simulink model "SF009A_DutyCycThermProtn"  (R2013b)
settings: Solver=FixedStepDiscrete  SolverMode=SingleTasking  StartTime=0.0  StopTime=1  FixedStep=0.1  RelTol=1e-3
undefined symbols (not defined in the file): AbsltTThermLimCnt, ARCHGLBPRM_100MILLISEC_SEC_F32, CTRLRANDCUTFLT_CNT_U08, CTRLRTFLT_CNT_U08, CUTFLT_CNT_U08, DITHERMLIM_MOTNWTMTR_F32, DutyCycExcddCnt, DutyCycThermProtnAbsltCtrlTTblX, DutyCycThermProtnAbsltCtrlTTqTblY, DutyCycThermProtnAbsltCuTTblX, DutyCycThermProtnAbsltCuTTqTblY, DutyCycThermProtnAbsltMotVelBreakPt, DutyCycThermProtnAbsltTTqSlewHiLim, DutyCycThermProtnAbsltTTqSlewLoLim, DutyCycThermProtnCtrlT, DutyCycThermProtnCtrlTSeln, DutyCycThermProtnDutyCycFildThd, DutyCycThermProtnIgnOffCtrlEna, DutyCycThermProtnIgnOffMsgWaitTi, DutyCycThermProtnLstTblValNonStall, DutyCycThermProtnLstTblValStall, DutyCycThermProtnMotPrTSeln, DutyCycThermProtnMplr1NonStallTblY, DutyCycThermProtnMplr1StallTblY, DutyCycThermProtnMplr2NonStallTblY, DutyCycThermProtnMplr2StallTblY, DutyCycThermProtnMplr3NonStallTblY, DutyCycThermProtnMplr3StallTblY, DutyCycThermProtnMplr4NonStallTblY, DutyCycThermProtnMplr4StallTblY, DutyCycThermProtnMplr5NonStallTblY, DutyCycThermProtnMplr5StallTblY, DutyCycThermProtnMplr6NonStallTblY, DutyCycThermProtnMplr6StallTblY, DutyCycThermProtnMplrTblX, DutyCycThermProtnMplrTSeln, DutyCycThermProtnSlowFilTSeln, DutyCycThermProtnThermLoadLimTblX, DutyCycThermProtnThermLoadLimTblY, DutyCycThermProtnTqCmdSlewDwn, DutyCycThermProtnTqCmdSlewUp, FILVALMIN_ULS_F32, IGNTIOFFTHD_CNT_F32, NODEBSTEP_CNT_U16, NtcSts1, NvmGetErrSts1, ONEPERC_ULS_F32, TAU3_SEC_F32, TAU4_SEC_F32, TAU5_SEC_F32, TAU6_SEC_F32, THERMLOADLIMTBLIDX_ULS_U08
libraries: FixdToFloat x13, Fil x12, simulink x11, NxtrLim x10, NxtrMath x8, FloatToFixd x6, NxtrMax x6, NxtrMin x4, NxtrAbslt x2, NxtrNvM x1
(part 4 of 6)

== system SF009A_DutyCycThermProtn/DutyCycThermProtn/DutyCycThermProtnPer1/TemperatureSelection/Mult36T_DiagcStsLimdTPrfmncDisabled ==
  MotMagT : Inport
  MotWidgT : Inport  Port=2
  Action Port : ActionPort  ActionType=else
  Calibration2 : Constant  RequirementInfo="{'linktype_rmi_doors' '0000a52a (/E-STEER Core/SubSystem Specifications/Application Functions/SF009A Thermal Duty Cycle Protection)' '#SF009A_144' 'true' 'REQ:  SF009A_144' '' } %GIDa_f0f24eda_9e7b_4d73_b7e4_5f6aa894dd73"  Value=DutyCycThermProtnMotPrTSeln
  CopyRight2 : Subsystem  Description=|  mask(Copyright Information){none=on}
      | Copyright info block.                                               
      |                                                                     
      | Place copyright information at the top of every subsystem in design.
      mask prompts: none "No parameters"
      mask help: Place copyright information at the top of every subsystem in design.
      mask Display:
      | NxtrConf = 'Nexteer Confidential';
      | 
      | sys = bdroot; %handle for the current model ("system")
      | first = get_param(sys,'Created');
      | first = first(end-3:end);  %year is last four digits
      | 
      | last = get_param(sys,'LastModifiedDate');
      | if isempty(last)
      |     last = datestr(now,'yyyy');
      | else
      |     last = last(end-3:end);
      | end
      | 
      | if strcmp(first,last)
      |     fprintf('%s -- Copyright %s Nexteer',NxtrConf,first)
      | else
      |     fprintf('%s -- %s%s- %s Nexteer',NxtrConf,char(169),first,last)
      | end
  If4 : If  RequirementInfo="{'linktype_rmi_doors' '0000a52a (/E-STEER Core/SubSystem Specifications/Application Functions/SF009A Thermal Duty Cycle Protection)' '#SF009A_144' 'true' 'REQ:  SF009A_144' '' } %GIDa_9a47a2e9_7f28_43d1_84f7_9c3425e558ba"  IfExpression=u1
  Merge4 : Merge  RequirementInfo="{'linktype_rmi_doors' '0000a52a (/E-STEER Core/SubSystem Specifications/Application Functions/SF009A Thermal Duty Cycle Protection)' '#SF009A_144' 'true' 'REQ:  SF009A_144' '' } %GIDa_e830a63c_d6ec_4209_a7ba_269af8b2217d"
  MotPrTSelnDisabled : Subsystem  RequirementInfo="{'linktype_rmi_doors' '0000a52a (/E-STEER Core/SubSystem Specifications/Application Functions/SF009A Thermal Duty Cycle Protection)' '#SF009A_144' 'true' 'REQ:  SF009A_144' '' } %GIDa_b554413f_6212_4f00_8e7a_d2a51ebc8c5c"  TreatAsAtomicUnit=on
  MotPrTSelnEnabled : Subsystem  RequirementInfo="{'linktype_rmi_doors' '0000a52a (/E-STEER Core/SubSystem Specifications/Application Functions/SF009A Thermal Duty Cycle Protection)' '#SF009A_144' 'true' 'REQ:  SF009A_144' '' } %GIDa_5495cb55_f8bc_4002_89d3_d2e432b2479b"  TreatAsAtomicUnit=on
  Mult36Temp : Outport
  wires:
  MotPrTSelnEnabled/1(Mult36) -> Merge4/1
  MotPrTSelnDisabled/1(Mult36) -> Merge4/2
  Calibration2/1 -> If4/1
  MotMagT/1 -> MotPrTSelnEnabled/1(MotMagT)
  MotWidgT/1 -> MotPrTSelnDisabled/1(MotWidgT)
  If4/1 -> MotPrTSelnEnabled/Action
  If4/2 -> MotPrTSelnDisabled/Action
  Merge4/1 -> Mult36Temp/1  "Mult36"

== system SF009A_DutyCycThermProtn/DutyCycThermProtn/DutyCycThermProtnPer1/TemperatureSelection/Mult36T_DiagcStsLimdTPrfmncEnabled ==
  Action Port : ActionPort  ActionType=then
  Calibration4 : Constant  RequirementInfo="{'linktype_rmi_doors' '0000a52a (/E-STEER Core/SubSystem Specifications/Application Functions/SF009A Thermal Duty Cycle Protection)' '#SF009A_144' 'true' 'REQ:  SF009A_144' '' } %GIDa_3ed4d287_d822_4a57_b7ce_3b57540e0243"  Value=DutyCycThermProtnCtrlT
  CopyRight2 : Subsystem  Description=|  mask(Copyright Information){none=on}
      | Copyright info block.                                               
      |                                                                     
      | Place copyright information at the top of every subsystem in design.
      mask prompts: none "No parameters"
      mask help: Place copyright information at the top of every subsystem in design.
      mask Display:
      | NxtrConf = 'Nexteer Confidential';
      | 
      | sys = bdroot; %handle for the current model ("system")
      | first = get_param(sys,'Created');
      | first = first(end-3:end);  %year is last four digits
      | 
      | last = get_param(sys,'LastModifiedDate');
      | if isempty(last)
      |     last = datestr(now,'yyyy');
      | else
      |     last = last(end-3:end);
      | end
      | 
      | if strcmp(first,last)
      |     fprintf('%s -- Copyright %s Nexteer',NxtrConf,first)
      | else
      |     fprintf('%s -- %s%s- %s Nexteer',NxtrConf,char(169),first,last)
      | end
  Mult36Temp : Outport
  wires:
  Calibration4/1 -> Mult36Temp/1

== system SF009A_DutyCycThermProtn/DutyCycThermProtn/DutyCycThermProtnPer1/TempratureLimiting/CopyRight2 ==

== system SF009A_DutyCycThermProtn/DutyCycThermProtn/DutyCycThermProtnPer1/TempratureLimiting/SetCtrlrAndCuTFltNtc ==
  Action Port : ActionPort  ActionType=then
  Constant23 : Constant  RequirementInfo="{'linktype_rmi_doors' '0000a52a (/E-STEER Core/SubSystem Specifications/Application Functions/SF009A Thermal Duty Cycle Protection)' '#SF009A_248' 'true' 'REQ:  SF009A_248' '' } %GIDa_eecd097f_77ad_4a7b_bdb8_19b5b9b4f39b"  Value=CTRLRANDCUTFLT_CNT_U08
  CopyRight2 : Subsystem  Description=|  mask(Copyright Information){none=on}
      | Copyright info block.                                               
      |                                                                     
      | Place copyright information at the top of every subsystem in design.
      mask prompts: none "No parameters"
      mask help: Place copyright information at the top of every subsystem in design.
      mask Display:
      | NxtrConf = 'Nexteer Confidential';
      | 
      | sys = bdroot; %handle for the current model ("system")
      | first = get_param(sys,'Created');
      | if(isempty(first))
      |     first = datestr(now,'yyyy');
      | else
      |     first = first(end-3:end);  %year is last four digits
      | end
      | 
      | last = get_param(sys,'LastModifiedDate');
      | if isempty(last)
      |     last = datestr(now,'yyyy');
      | else
      |     last = last(end-3:end);
      | end
      | 
      | if strcmp(first,last)
      |     fprintf('%s -- Copyright %s Nexteer',NxtrConf,first)
      | else
      |     fprintf('%s -- %s%s- %s Nexteer',NxtrConf,char(169),first,last)
      | end
  Enumerated Constant7 : simulink/Sources/Enumerated Constant  RequirementInfo="{'linktype_rmi_doors' '0000a52a (/E-STEER Core/SubSystem Specifications/Application Functions/SF009A Thermal Duty Cycle Protection)' '#SF009A_248' 'true' 'REQ:  SF009A_248' '' } %GIDa_403c372b_2528_42cf_824a_3c84739cf9bb"  OutDataTypeStr=Enum: NtcSts1  Value=NtcSts1.NTCSTS_FAILD  SampleTime=inf
  Out1 : Outport
  Out2 : Outport  Port=2
  wires:
  Constant23/1 -> Out1/1
  Enumerated Constant7/1 -> Out2/1

== system SF009A_DutyCycThermProtn/DutyCycThermProtn/DutyCycThermProtnPer1/TempratureLimiting/SetCtrlrTFltNtc ==
  Action Port : ActionPort  ActionType=elseif
  Constant25 : Constant  RequirementInfo="{'linktype_rmi_doors' '0000a52a (/E-STEER Core/SubSystem Specifications/Application Functions/SF009A Thermal Duty Cycle Protection)' '#SF009A_248' 'true' 'REQ:  SF009A_248' '' } %GIDa_45d14f2e_33e7_442d_980c_33b708f78f49"  Value=CTRLRTFLT_CNT_U08
  CopyRight2 : Subsystem  Description=|  mask(Copyright Information){none=on}
      | Copyright info block.                                               
      |                                                                     
      | Place copyright information at the top of every subsystem in design.
      mask prompts: none "No parameters"
      mask help: Place copyright information at the top of every subsystem in design.
      mask Display:
      | NxtrConf = 'Nexteer Confidential';
      | 
      | sys = bdroot; %handle for the current model ("system")
      | first = get_param(sys,'Created');
      | if(isempty(first))
      |     first = datestr(now,'yyyy');
      | else
      |     first = first(end-3:end);  %year is last four digits
      | end
      | 
      | last = get_param(sys,'LastModifiedDate');
      | if isempty(last)
      |     last = datestr(now,'yyyy');
      | else
      |     last = last(end-3:end);
      | end
      | 
      | if strcmp(first,last)
      |     fprintf('%s -- Copyright %s Nexteer',NxtrConf,first)
      | else
      |     fprintf('%s -- %s%s- %s Nexteer',NxtrConf,char(169),first,last)
      | end
  Enumerated Constant13 : simulink/Sources/Enumerated Constant  RequirementInfo="{'linktype_rmi_doors' '0000a52a (/E-STEER Core/SubSystem Specifications/Application Functions/SF009A Thermal Duty Cycle Protection)' '#SF009A_248' 'true' 'REQ:  SF009A_248' '' } %GIDa_05e09b87_7e7f_4e95_9fb1_18c3f562049e"  OutDataTypeStr=Enum: NtcSts1  Value=NtcSts1.NTCSTS_FAILD  SampleTime=inf
  Out1 : Outport
  Out2 : Outport  Port=2
  wires:
  Enumerated Constant13/1 -> Out2/1
  Constant25/1 -> Out1/1

== system SF009A_DutyCycThermProtn/DutyCycThermProtn/DutyCycThermProtnPer1/TempratureLimiting/SetCuTFltNtc ==
  Action Port : ActionPort  ActionType=elseif
  Constant27 : Constant  RequirementInfo="{'linktype_rmi_doors' '0000a52a (/E-STEER Core/SubSystem Specifications/Application Functions/SF009A Thermal Duty Cycle Protection)' '#SF009A_248' 'true' 'REQ:  SF009A_248' '' } %GIDa_5abe4f1d_a9ab_402f_b899_5b241470b6cc"  Value=CUTFLT_CNT_U08
  CopyRight2 : Subsystem  Description=|  mask(Copyright Information){none=on}
      | Copyright info block.                                               
      |                                                                     
      | Place copyright information at the top of every subsystem in design.
      mask prompts: none "No parameters"
      mask help: Place copyright information at the top of every subsystem in design.
      mask Display:
      | NxtrConf = 'Nexteer Confidential';
      | 
      | sys = bdroot; %handle for the current model ("system")
      | first = get_param(sys,'Created');
      | if(isempty(first))
      |     first = datestr(now,'yyyy');
      | else
      |     first = first(end-3:end);  %year is last four digits
      | end
      | 
      | last = get_param(sys,'LastModifiedDate');
      | if isempty(last)
      |     last = datestr(now,'yyyy');
      | else
      |     last = last(end-3:end);
      | end
      | 
      | if strcmp(first,last)
      |     fprintf('%s -- Copyright %s Nexteer',NxtrConf,first)
      | else
      |     fprintf('%s -- %s%s- %s Nexteer',NxtrConf,char(169),first,last)
      | end
  Enumerated Constant15 : simulink/Sources/Enumerated Constant  RequirementInfo="{'linktype_rmi_doors' '0000a52a (/E-STEER Core/SubSystem Specifications/Application Functions/SF009A Thermal Duty Cycle Protection)' '#SF009A_248' 'true' 'REQ:  SF009A_248' '' } %GIDa_13f324ce_9b74_4823_8d4c_43ce25139662"  OutDataTypeStr=Enum: NtcSts1  Value=NtcSts1.NTCSTS_FAILD  SampleTime=inf
  Out1 : Outport
  Out2 : Outport  Port=2
  wires:
  Constant27/1 -> Out1/1
  Enumerated Constant15/1 -> Out2/1

== system SF009A_DutyCycThermProtn/DutyCycThermProtn/DutyCycThermProtnPer1/TempratureLimiting/SetNtc ==
  NtcNr : Inport
  NtcStInfo : Inport  Port=2
  NtcSts : Inport  Port=3
  DebStep : Inport  Port=4
  CopyRight2 : Subsystem  Description=|  mask(Copyright Information){none=on}
      | Copyright info block.                                               
      |                                                                     
      | Place copyright information at the top of every subsystem in design.
      mask prompts: none "No parameters"
      mask help: Place copyright information at the top of every subsystem in design.
      mask Display:
      | NxtrConf = 'Nexteer Confidential';
      | 
      | sys = bdroot; %handle for the current model ("system")
      | first = get_param(sys,'Created');
      | first = first(end-3:end);  %year is last four digits
      | 
      | last = get_param(sys,'LastModifiedDate');
      | if isempty(last)
      |     last = datestr(now,'yyyy');
      | else
      |     last = last(end-3:end);
      | end
      | 
      | if strcmp(first,last)
      |     fprintf('%s -- Copyright %s Nexteer',NxtrConf,first)
      | else
      |     fprintf('%s -- %s%s- %s Nexteer',NxtrConf,char(169),first,last)
      | end
  SetNtcSts : Subsystem  RequirementInfo={} %GIDa_f4639b12_c119_4531_89d0_f202df3b56bb
  wires:
  NtcStInfo/1 -> SetNtcSts/2(NtcStInfo)
  NtcSts/1 -> SetNtcSts/3(NtcSts)
  NtcNr/1 -> SetNtcSts/1(NtcNr)
  DebStep/1 -> SetNtcSts/4(DebStep)

== system SF009A_DutyCycThermProtn/DutyCycThermProtn/DutyCycThermProtnPer1/TempratureLimiting/SetPassdNtc ==
  Action Port : ActionPort  ActionType=else
  Constant9 : Constant  RequirementInfo="{'linktype_rmi_doors' '0000a52a (/E-STEER Core/SubSystem Specifications/Application Functions/SF009A Thermal Duty Cycle Protection)' '#SF009A_248' 'true' 'REQ:  SF009A_248' '' } %GIDa_52bd9a26_a3c7_4cca_a4b7_c0bf150f71af"  Value=0  OutDataTypeStr=uint8
      settings: AttributesFormatString=%<OutDataTypeStr>
  CopyRight2 : Subsystem  Description=|  mask(Copyright Information){none=on}
      | Copyright info block.                                               
      |                                                                     
      | Place copyright information at the top of every subsystem in design.
      mask prompts: none "No parameters"
      mask help: Place copyright information at the top of every subsystem in design.
      mask Display:
      | NxtrConf = 'Nexteer Confidential';
      | 
      | sys = bdroot; %handle for the current model ("system")
      | first = get_param(sys,'Created');
      | if(isempty(first))
      |     first = datestr(now,'yyyy');
      | else
      |     first = first(end-3:end);  %year is last four digits
      | end
      | 
      | last = get_param(sys,'LastModifiedDate');
      | if isempty(last)
      |     last = datestr(now,'yyyy');
      | else
      |     last = last(end-3:end);
      | end
      | 
      | if strcmp(first,last)
      |     fprintf('%s -- Copyright %s Nexteer',NxtrConf,first)
      | else
      |     fprintf('%s -- %s%s- %s Nexteer',NxtrConf,char(169),first,last)
      | end
  Enumerated Constant2 : simulink/Sources/Enumerated Constant  RequirementInfo="{'linktype_rmi_doors' '0000a52a (/E-STEER Core/SubSystem Specifications/Application Functions/SF009A Thermal Duty Cycle Protection)' '#SF009A_248' 'true' 'REQ:  SF009A_248' '' } %GIDa_418efcac_b2fe_4078_9302_4b7835e96a36"  OutDataTypeStr=Enum: NtcSts1  Value=NtcSts1.NTCSTS_PASSD  SampleTime=inf
  Out1 : Outport
  Out2 : Outport  Port=2
  wires:
  Enumerated Constant2/1 -> Out2/1
  Constant9/1 -> Out1/1

== system SF009A_DutyCycThermProtn/DutyCycThermProtn/DutyCycThermProtnPer1/ThermalLimitStatus/CopyRight2 ==

== system SF009A_DutyCycThermProtn/DutyCycThermProtn/DutyCycThermProtnPer1/ThermalLimitStatus/DutyCycThermProtnDisabled ==
  Action Port : ActionPort  ActionType=then
  CopyRight2 : Subsystem  Description=|  mask(Copyright Information){none=on}
      | Copyright info block.                                               
      |                                                                     
      | Place copyright information at the top of every subsystem in design.
      mask prompts: none "No parameters"
      mask help: Place copyright information at the top of every subsystem in design.
      mask Display:
      | NxtrConf = 'Nexteer Confidential';
      | 
      | sys = bdroot; %handle for the current model ("system")
      | first = get_param(sys,'Created');
      | first = first(end-3:end);  %year is last four digits
      | 
      | last = get_param(sys,'LastModifiedDate');
      | if isempty(last)
      |     last = datestr(now,'yyyy');
      | else
      |     last = last(end-3:end);
      | end
      | 
      | if strcmp(first,last)
      |     fprintf('%s -- Copyright %s Nexteer',NxtrConf,first)
      | else
      |     fprintf('%s -- %s%s- %s Nexteer',NxtrConf,char(169),first,last)
      | end
  D_DEFEATTHERMALLIMITPERC_ULS : Constant  Value=0  OutDataTypeStr=Inherit: Inherit via back propagation
  ThermRednFac : Outport
  wires:
  D_DEFEATTHERMALLIMITPERC_ULS/1 -> ThermRednFac/1

== system SF009A_DutyCycThermProtn/DutyCycThermProtn/DutyCycThermProtnPer1/ThermalLimitStatus/DutyCycThermProtnEnabled  ==
  note: Calculate the percent reduction in allowable output.
  ThermLim : Inport
  Action Port : ActionPort  ActionType=else
  Constant : Constant  RequirementInfo="{'linktype_rmi_doors' '0000a52a (/E-STEER Core/SubSystem Specifications/Application Functions/SF009A Thermal Duty Cycle Protection)' '#SF009A_235' 'true' 'REQ:  SF009A_235' '' } %GIDa_16531b45_897e_4dc4_b513_05ce1dab48c2"  Value=0
  CopyRight2 : Subsystem  Description=|  mask(Copyright Information){none=on}
      | Copyright info block.                                               
      |                                                                     
      | Place copyright information at the top of every subsystem in design.
      mask prompts: none "No parameters"
      mask help: Place copyright information at the top of every subsystem in design.
      mask Display:
      | NxtrConf = 'Nexteer Confidential';
      | 
      | sys = bdroot; %handle for the current model ("system")
      | first = get_param(sys,'Created');
      | first = first(end-3:end);  %year is last four digits
      | 
      | last = get_param(sys,'LastModifiedDate');
      | if isempty(last)
      |     last = datestr(now,'yyyy');
      | else
      |     last = last(end-3:end);
      | end
      | 
      | if strcmp(first,last)
      |     fprintf('%s -- Copyright %s Nexteer',NxtrConf,first)
      | else
      |     fprintf('%s -- %s%s- %s Nexteer',NxtrConf,char(169),first,last)
      | end
  D_1PERC_ULS : Constant  RequirementInfo="{'linktype_rmi_doors' '0000a52a (/E-STEER Core/SubSystem Specifications/Application Functions/SF009A Thermal Duty Cycle Protection)' '#SF009A_235' 'true' 'REQ:  SF009A_235' '' } %GIDa_93aa9e31_1bb6_4aa8_990d_71db7a9b41ac"  Value=ONEPERC_ULS_F32
  D_ONE_ULS : Constant  OutDataTypeStr=Inherit: Inherit via back propagation
  "D_ONE_ULS " : Constant  OutDataTypeStr=Inherit: Inherit via back propagation
  Data Store Write : DataStoreWrite  DataStoreName=dDutyCycThermProtnThermLoadLimTblYVal
  Divide : Product  RequirementInfo="{'linktype_rmi_doors' '0000a52a (/E-STEER Core/SubSystem Specifications/Application Functions/SF009A Thermal Duty Cycle Protection)' '#SF009A_235' 'true' 'REQ:  SF009A_235' '' } %GIDa_2859e81a_9c0b_47c3_a3e7_7b6ba932546b"  Inputs=*/
  FixdToFloat_f32_u16 : FixdToFloat/FixdToFloat_f32_u16  RequirementInfo="{'linktype_rmi_doors' '0000a52a (/E-STEER Core/SubSystem Specifications/Application Functions/SF009A Thermal Duty Cycle Protection)' '#SF009A_235' 'true' 'REQ:  SF009A_235' '' } %GIDa_1b62b4bf_ccb3_4bc2_887e_098fc4042f26"  Param1=7
  Max_f32 : NxtrMax/Max_f32  RequirementInfo="{'linktype_rmi_doors' '0000a52a (/E-STEER Core/SubSystem Specifications/Application Functions/SF009A Thermal Duty Cycle Protection)' '#SF009A_235' 'true' 'REQ:  SF009A_235' '' } %GIDa_7c8fb2af_5fc5_4bef_aca3_69542eb779f3"  SFunctionSpec=single y1 = Max_f32(single u1, single u2)
      settings: AttributesFormatString=%<Name>
  Min_f32 : NxtrMin/Min_f32  SFunctionSpec=single y1 = Min_f32(single u1, single u2)
      settings: AttributesFormatString=%<Name>
  Selector : Selector  RequirementInfo="{'linktype_rmi_doors' '0000a52a (/E-STEER Core/SubSystem Specifications/Application Functions/SF009A Thermal Duty Cycle Protection)' '#SF009A_235' 'true' 'REQ:  SF009A_235' '' } %GIDa_638fe986_5675_4fa6_a0db_cf353cf2df77"  IndexMode=Zero-based  InputPortWidth=8  IndexOptions=Index vector (port)  Indices=[1 3]  OutputSizes=1
  Subtract : Sum  Inputs=+-  OutDataTypeStr=Inherit: Inherit via back propagation
  const1 : Constant  RequirementInfo="{'linktype_rmi_doors' '0000a52a (/E-STEER Core/SubSystem Specifications/Application Functions/SF009A Thermal Duty Cycle Protection)' '#SF009A_235' 'true' 'REQ:  SF009A_235' '' } %GIDa_bc470105_196c_4f91_a524_dc4b976ba41f"  Value=DutyCycThermProtnThermLoadLimTblY
  ThermRednFac : Outport
  wires:
  ThermLim/1 -> Divide/1
  D_1PERC_ULS/1 -> Max_f32/2
  Max_f32/1 -> Divide/2, Data Store Write/1  "DivFactor"
  Divide/1 -> Min_f32/1
  Min_f32/1 -> Subtract/2
  D_ONE_ULS/1 -> Subtract/1
  "D_ONE_ULS "/1 -> Min_f32/2
  Subtract/1 -> ThermRednFac/1
  const1/1 -> Selector/1
  Constant/1 -> Selector/2
  Selector/1 -> FixdToFloat_f32_u16/1
  FixdToFloat_f32_u16/1 -> Max_f32/1

== system SF009A_DutyCycThermProtn/DutyCycThermProtn/DutyCycThermProtnPer1/ThermalLimitStatus/MaxoutLimiting ==
  note: The if trigger of DutyCycThermProtnDi logic is changed
  note: Since the NTC set to Pass or Fail directly, the debounce step does not matter.
  note: Determine whether the output is being limited or not.
  Maxout : Inport  RequirementInfo={} %GIDa_c9033dbb_9425_41b9_afac_070c8cac5788
  DutyCycThermProtnDi : Inport  Port=2
  Calibration : Constant  RequirementInfo="{'linktype_rmi_doors' '0000a52a (/E-STEER Core/SubSystem Specifications/Application Functions/SF009A Thermal Duty Cycle Protection)' '#SF009A_143' 'true' 'REQ:  SF009A_143' '' } %GIDa_c2c776cc_23eb_4dd4_af42_dded3d6af954"  Value=DutyCycThermProtnDutyCycFildThd
  Calibration1 : Constant  RequirementInfo="{'linktype_rmi_doors' '0000a52a (/E-STEER Core/SubSystem Specifications/Application Functions/SF009A Thermal Duty Cycle Protection)' '#SF009A_143' 'true' 'REQ:  SF009A_143' '' } %GIDa_d01dd759_96c6_4cf8_a92b_ce6e4a929ac5"  Value=0  OutDataTypeStr=uint8
      settings: AttributesFormatString=%<OutDataTypeStr>
  Calibration2 : Constant  RequirementInfo="{'linktype_rmi_doors' '0000a52a (/E-STEER Core/SubSystem Specifications/Application Functions/SF009A Thermal Duty Cycle Protection)' '#SF009A_143' 'true' 'REQ:  SF009A_143' '' } %GIDa_4165ff0d_ee55_4ed1_bff8_c9ab25f540fd"  Value=NODEBSTEP_CNT_U16
  Calibration3 : Constant  RequirementInfo="{'linktype_rmi_doors' '0000a52a (/E-STEER Core/SubSystem Specifications/Application Functions/SF009A Thermal Duty Cycle Protection)' '#SF009A_287' 'true' 'REQ:  SF009A_287' '' } %GIDa_9e49d4ad_c406_45fe_8285_ce8bcc9ea311"  Value=DutyCycExcddCnt
  Calibration4 : Constant  RequirementInfo="{'linktype_rmi_doors' '0000a52a (/E-STEER Core/SubSystem Specifications/Application Functions/SF009A Thermal Duty Cycle Protection)' '#SF009A_287' 'true' 'REQ:  SF009A_287' '' } %GIDa_909d4211_68a2_485e_8009_556c9d2ea048"  Value=0  OutDataTypeStr=uint8
      settings: AttributesFormatString=%<OutDataTypeStr>
  Calibration5 : Constant  RequirementInfo="{'linktype_rmi_doors' '0000a52a (/E-STEER Core/SubSystem Specifications/Application Functions/SF009A Thermal Duty Cycle Protection)' '#SF009A_287' 'true' 'REQ:  SF009A_287' '' } %GIDa_3197ff62_cd6c_4cc1_97de_b408274b636f"  Value=NODEBSTEP_CNT_U16
  Calibration6 : Constant  RequirementInfo="{'linktype_rmi_doors' '0000a52a (/E-STEER Core/SubSystem Specifications/Application Functions/SF009A Thermal Duty Cycle Protection)' '#SF009A_143' 'true' 'REQ:  SF009A_143' '' } %GIDa_aad2f3e7_35aa_44c1_bde4_89a84bfb87a8"  Value=DutyCycExcddCnt
  CopyRight2 : Subsystem  Description=|  mask(Copyright Information){none=on}
      | Copyright info block.                                               
      |                                                                     
      | Place copyright information at the top of every subsystem in design.
      mask prompts: none "No parameters"
      mask help: Place copyright information at the top of every subsystem in design.
      mask Display:
      | NxtrConf = 'Nexteer Confidential';
      | 
      | sys = bdroot; %handle for the current model ("system")
      | first = get_param(sys,'Created');
      | first = first(end-3:end);  %year is last four digits
      | 
      | last = get_param(sys,'LastModifiedDate');
      | if isempty(last)
      |     last = datestr(now,'yyyy');
      | else
      |     last = last(end-3:end);
      | end
      | 
      | if strcmp(first,last)
      |     fprintf('%s -- Copyright %s Nexteer',NxtrConf,first)
      | else
      |     fprintf('%s -- %s%s- %s Nexteer',NxtrConf,char(169),first,last)
      | end
  If : If  RequirementInfo="{'linktype_rmi_doors' '0000a52a (/E-STEER Core/SubSystem Specifications/Application Functions/SF009A Thermal Duty Cycle Protection)' '#SF009A_143' 'true' 'REQ:  SF009A_143' '' ; 'linktype_rmi_doors' '0000a52a (/E-STEER Core/SubSystem Specifications/Application Functions/SF009A Thermal Duty Cycle Protection)' '#SF009A_287' 'true' 'REQ:  SF009A_287' '' } %GIDa_931709a6_5c4c_4b44_801e_2d8d92c465f4"  IfExpression=~u1
  Logical Operator : Logic  RequirementInfo="{'linktype_rmi_doors' '0000a52a (/E-STEER Core/SubSystem Specifications/Application Functions/SF009A Thermal Duty Cycle Protection)' '#SF009A_143' 'true' 'REQ:  SF009A_143' '' } %GIDa_124c66df_9600_46ad_b4d3_628bc6f7d811"  AllPortsSameDT=off  OutDataTypeStr=boolean
  Logical Operator1 : Logic  RequirementInfo="{'linktype_rmi_doors' '0000a52a (/E-STEER Core/SubSystem Specifications/Application Functions/SF009A Thermal Duty Cycle Protection)' '#SF009A_143' 'true' 'REQ:  SF009A_143' '' } %GIDa_4463f4d1_0634_48fe_8fb9_d68ce118fb92"  Operator=NOT  Inputs=1  AllPortsSameDT=off  OutDataTypeStr=boolean
  NtcSts : simulink/Sources/Enumerated Constant  RequirementInfo="{'linktype_rmi_doors' '0000a52a (/E-STEER Core/SubSystem Specifications/Application Functions/SF009A Thermal Duty Cycle Protection)' '#SF009A_287' 'true' 'REQ:  SF009A_287' '' } %GIDa_aec53b8e_e8f2_420b_a9a6_daaf6f3004da"  OutDataTypeStr=Enum: NtcSts1  Value=NtcSts1.NTCSTS_PASSD  SampleTime=inf
  NtcSts1 : simulink/Sources/Enumerated Constant  RequirementInfo="{'linktype_rmi_doors' '0000a52a (/E-STEER Core/SubSystem Specifications/Application Functions/SF009A Thermal Duty Cycle Protection)' '#SF009A_143' 'true' 'REQ:  SF009A_143' '' } %GIDa_94f0ec75_311c_40ec_9c65_7fd82f034551"  OutDataTypeStr=Enum: NtcSts1  Value=NtcSts1.NTCSTS_FAILD  SampleTime=inf
  Relational Operator : RelationalOperator  RequirementInfo="{'linktype_rmi_doors' '0000a52a (/E-STEER Core/SubSystem Specifications/Application Functions/SF009A Thermal Duty Cycle Protection)' '#SF009A_143' 'true' 'REQ:  SF009A_143' '' } %GIDa_a3e6ed02_380b_485a_84a6_acfe969451a8"  OutDataTypeStr=boolean
  SetNtcFail : Subsystem  RequirementInfo="{'linktype_rmi_doors' '0000a52a (/E-STEER Core/SubSystem Specifications/Application Functions/SF009A Thermal Duty Cycle Protection)' '#SF009A_143' 'true' 'REQ:  SF009A_143' '' } %GIDa_819066fa_129b_472c_8396_25b2b8bd49d8"  TreatAsAtomicUnit=on  mask(SetNTC){}
      mask help: SetNTC library block
  SetNtcPass : Subsystem  RequirementInfo="{'linktype_rmi_doors' '0000a52a (/E-STEER Core/SubSystem Specifications/Application Functions/SF009A Thermal Duty Cycle Protection)' '#SF009A_287' 'true' 'REQ:  SF009A_287' '' } %GIDa_4c5cba3c_7974_4ea9_a664_d9a08749424d"  TreatAsAtomicUnit=on  mask(SetNTC){}
      mask help: SetNTC library block
  wires:
  Calibration/1 -> Relational Operator/2
  Relational Operator/1 -> Logical Operator/1  "true_ntc_sts"
  Calibration5/1 -> SetNtcPass/4(DebStep)
  If/2 -> SetNtcFail/Action
  If/1 -> SetNtcPass/Action
  Calibration3/1 -> SetNtcPass/1(NtcNr)
  NtcSts/1 -> SetNtcPass/3(NtcSts)
  NtcSts1/1 -> SetNtcFail/3(NtcSts)
  Calibration2/1 -> SetNtcFail/4(DebStep)
  Calibration6/1 -> SetNtcFail/1(NtcNr)
  Calibration1/1 -> SetNtcFail/2(NtcStInfo)
  Calibration4/1 -> SetNtcPass/2(NtcStInfo)
  Maxout/1 -> Relational Operator/1
  DutyCycThermProtnDi/1 -> Logical Operator1/1
  Logical Operator1/1 -> Logical Operator/2
  Logical Operator/1 -> If/1

== system SF009A_DutyCycThermProtn/DutyCycThermProtn/DutyCycThermProtnPer1/ThermalLimitStatus/ThermLim_DutyCycThermProtnDisabled ==
  AbsTempLimitSlew : Inport
  Action Port : ActionPort  ActionType=then
  CopyRight2 : Subsystem  Description=|  mask(Copyright Information){none=on}
      | Copyright info block.                                               
      |                                                                     
      | Place copyright information at the top of every subsystem in design.
      mask prompts: none "No parameters"
      mask help: Place copyright information at the top of every subsystem in design.
      mask Display:
      | NxtrConf = 'Nexteer Confidential';
      | 
      | sys = bdroot; %handle for the current model ("system")
      | first = get_param(sys,'Created');
      | first = first(end-3:end);  %year is last four digits
      | 
      | last = get_param(sys,'LastModifiedDate');
      | if isempty(last)
      |     last = datestr(now,'yyyy');
      | else
      |     last = last(end-3:end);
      | end
      | 
      | if strcmp(first,last)
      |     fprintf('%s -- Copyright %s Nexteer',NxtrConf,first)
      | else
      |     fprintf('%s -- %s%s- %s Nexteer',NxtrConf,char(169),first,last)
      | end
  D_DEFEATTHERMLLIMIT_MTRNM : Constant  RequirementInfo="{'linktype_rmi_doors' '0000a52a (/E-STEER Core/SubSystem Specifications/Application Functions/SF009A Thermal Duty Cycle Protection)' '#SF009A_233' 'true' 'REQ:  SF009A_233' '' } %GIDa_1cb6d24b_5473_47d9_a778_4e29cc776369"  Value=DITHERMLIM_MOTNWTMTR_F32
  Min_f32 : NxtrMin/Min_f32  RequirementInfo="{'linktype_rmi_doors' '0000a52a (/E-STEER Core/SubSystem Specifications/Application Functions/SF009A Thermal Duty Cycle Protection)' '#SF009A_233' 'true' 'REQ:  SF009A_233' '' } %GIDa_ed82a7aa_ec0a_4a98_b588_9880534c0008"  SFunctionSpec=single y1 = Min_f32(single u1, single u2)
  DftThermLmt : Outport
  wires:
  AbsTempLimitSlew/1 -> Min_f32/1
  D_DEFEATTHERMLLIMIT_MTRNM/1 -> Min_f32/2
  Min_f32/1 -> DftThermLmt/1

== system SF009A_DutyCycThermProtn/DutyCycThermProtn/DutyCycThermProtnPer1/ThermalLimitStatus/ThermLim_DutyCycThermProtnEnabled ==
  AbsTempLimitSlew : Inport
  ThermalLoadLmt : Inport  Port=2
  Action Port : ActionPort  ActionType=else
  CopyRight2 : Subsystem  Description=|  mask(Copyright Information){none=on}
      | Copyright info block.                                               
      |                                                                     
      | Place copyright information at the top of every subsystem in design.
      mask prompts: none "No parameters"
      mask help: Place copyright information at the top of every subsystem in design.
      mask Display:
      | NxtrConf = 'Nexteer Confidential';
      | 
      | sys = bdroot; %handle for the current model ("system")
      | first = get_param(sys,'Created');
      | first = first(end-3:end);  %year is last four digits
      | 
      | last = get_param(sys,'LastModifiedDate');
      | if isempty(last)
      |     last = datestr(now,'yyyy');
      | else
      |     last = last(end-3:end);
      | end
      | 
      | if strcmp(first,last)
      |     fprintf('%s -- Copyright %s Nexteer',NxtrConf,first)
      | else
      |     fprintf('%s -- %s%s- %s Nexteer',NxtrConf,char(169),first,last)
      | end
  Min_f1 : NxtrMin/Min_f32  RequirementInfo="{'linktype_rmi_doors' '0000a52a (/E-STEER Core/SubSystem Specifications/Application Functions/SF009A Thermal Duty Cycle Protection)' '#SF009A_232' 'true' 'REQ:  SF009A_232' '' } %GIDa_482469eb_3d25_4d81_9a4e_bd867fccbbc0"  SFunctionSpec=single y1 = Min_f32(single u1, single u2)
  ThermalLimit_Prelim : Outport
  wires:
  AbsTempLimitSlew/1 -> Min_f1/2
  ThermalLoadLmt/1 -> Min_f1/1
  Min_f1/1 -> ThermalLimit_Prelim/1

== system SF009A_DutyCycThermProtn/DutyCycThermProtn/DutyCycThermProtnInit1/PowerOnTasks/DefaultIgnOffTime/CopyRight2 ==

== system SF009A_DutyCycThermProtn/DutyCycThermProtn/DutyCycThermProtnInit1/PowerOnTasks/InputIgnOffTime/CopyRight2 ==

== system SF009A_DutyCycThermProtn/DutyCycThermProtn/DutyCycThermProtnInit1/PowerOnTasks/InputIgnOffTime/Filt3ExpDecay ==
  IgnTimeOffSel : Inport  RequirementInfo="{'linktype_rmi_doors' '0000a52a (/E-STEER Core/SubSystem Specifications/Application Functions/SF009A Thermal Duty Cycle Protection)' '#SF009A_285' 'true' 'REQ:  SF009A_285' '' } %GIDa_5c5cb044_26c8_4dbf_bfdb_5ff65517aeea"
  FiltSVOrg : Inport  RequirementInfo="{'linktype_rmi_doors' '0000a52a (/E-STEER Core/SubSystem Specifications/Application Functions/SF009A Thermal Duty Cycle Protection)' '#SF009A_285' 'true' 'REQ:  SF009A_285' '' } %GIDa_91a7a242_3564_4b75_930d_3be3ef1f28fd"  Port=2
  CopyRight2 : Subsystem  Description=|  mask(Copyright Information){none=on}
      | Copyright info block.                                               
      |                                                                     
      | Place copyright information at the top of every subsystem in design.
      mask prompts: none "No parameters"
      mask help: Place copyright information at the top of every subsystem in design.
      mask Display:
      | NxtrConf = 'Nexteer Confidential';
      | 
      | sys = bdroot; %handle for the current model ("system")
      | first = get_param(sys,'Created');
      | first = first(end-3:end);  %year is last four digits
      | 
      | last = get_param(sys,'LastModifiedDate');
      | if isempty(last)
      |     last = datestr(now,'yyyy');
      | else
      |     last = last(end-3:end);
      | end
      | 
      | if strcmp(first,last)
      |     fprintf('%s -- Copyright %s Nexteer',NxtrConf,first)
      | else
      |     fprintf('%s -- %s%s- %s Nexteer',NxtrConf,char(169),first,last)
      | end
  Exp_f32 : NxtrMath/Exp_f32  RequirementInfo="{'linktype_rmi_doors' '0000a52a (/E-STEER Core/SubSystem Specifications/Application Functions/SF009A Thermal Duty Cycle Protection)' '#SF009A_285' 'true' 'REQ:  SF009A_285' '' } %GIDa_7883efea_e5ae_4044_b7ed_02762036b56f"  SFunctionSpec=single y1 = Exp_f32(single u1)  ShowSpec=on
      settings: AttributesFormatString=%<MaskType>
  Gain : Gain  RequirementInfo="{'linktype_rmi_doors' '0000a52a (/E-STEER Core/SubSystem Specifications/Application Functions/SF009A Thermal Duty Cycle Protection)' '#SF009A_285' 'true' 'REQ:  SF009A_285' '' } %GIDa_88cc6e5b_9aec_42fe_9fe2_a5cfa1021eda"  Gain=-1
  Product1 : Product  RequirementInfo="{'linktype_rmi_doors' '0000a52a (/E-STEER Core/SubSystem Specifications/Application Functions/SF009A Thermal Duty Cycle Protection)' '#SF009A_285' 'true' 'REQ:  SF009A_285' '' } %GIDa_0fcfcda3_a01a_4d7a_af05_1e45f2a4ef74"  RndMeth=Zero
  Product2 : Product  RequirementInfo="{'linktype_rmi_doors' '0000a52a (/E-STEER Core/SubSystem Specifications/Application Functions/SF009A Thermal Duty Cycle Protection)' '#SF009A_285' 'true' 'REQ:  SF009A_285' '' } %GIDa_261a80b6_5869_428e_8277_22821d348308"  Inputs=*/  RndMeth=Zero
  Tau : Constant  RequirementInfo="{'linktype_rmi_doors' '0000a52a (/E-STEER Core/SubSystem Specifications/Application Functions/SF009A Thermal Duty Cycle Protection)' '#SF009A_285' 'true' 'REQ:  SF009A_285' '' } %GIDa_03bc81ed_1d96_46ca_851c_5da21a8f4976"  Value=TAU3_SEC_F32
  FiltSV : Outport  RequirementInfo="{'linktype_rmi_doors' '0000a52a (/E-STEER Core/SubSystem Specifications/Application Functions/SF009A Thermal Duty Cycle Protection)' '#SF009A_285' 'true' 'REQ:  SF009A_285' '' } %GIDa_bdc8e6b7_90e9_4d60_8279_bf082cc585c6"
  wires:
  FiltSVOrg/1 -> Product1/2
  Product1/1 -> FiltSV/1
  IgnTimeOffSel/1 -> Gain/1
  Tau/1 -> Product2/2
  Exp_f32/1 -> Product1/1
  Gain/1 -> Product2/1
  Product2/1 -> Exp_f32/1

== system SF009A_DutyCycThermProtn/DutyCycThermProtn/DutyCycThermProtnInit1/PowerOnTasks/InputIgnOffTime/Filt4ExpDecay ==
  IgnTimeOffSel : Inport  RequirementInfo="{'linktype_rmi_doors' '0000a52a (/E-STEER Core/SubSystem Specifications/Application Functions/SF009A Thermal Duty Cycle Protection)' '#SF009A_285' 'true' 'REQ:  SF009A_285' '' } %GIDa_7550d9c9_f333_4982_a7f0_be5fb272d54b"
  FiltSVOrg : Inport  RequirementInfo="{'linktype_rmi_doors' '0000a52a (/E-STEER Core/SubSystem Specifications/Application Functions/SF009A Thermal Duty Cycle Protection)' '#SF009A_285' 'true' 'REQ:  SF009A_285' '' } %GIDa_0ac67eff_405d_4d9d_b637_6c1188d91fb4"  Port=2
  CopyRight2 : Subsystem  Description=|  mask(Copyright Information){none=on}
      | Copyright info block.                                               
      |                                                                     
      | Place copyright information at the top of every subsystem in design.
      mask prompts: none "No parameters"
      mask help: Place copyright information at the top of every subsystem in design.
      mask Display:
      | NxtrConf = 'Nexteer Confidential';
      | 
      | sys = bdroot; %handle for the current model ("system")
      | first = get_param(sys,'Created');
      | first = first(end-3:end);  %year is last four digits
      | 
      | last = get_param(sys,'LastModifiedDate');
      | if isempty(last)
      |     last = datestr(now,'yyyy');
      | else
      |     last = last(end-3:end);
      | end
      | 
      | if strcmp(first,last)
      |     fprintf('%s -- Copyright %s Nexteer',NxtrConf,first)
      | else
      |     fprintf('%s -- %s%s- %s Nexteer',NxtrConf,char(169),first,last)
      | end
  Exp_f32 : NxtrMath/Exp_f32  RequirementInfo="{'linktype_rmi_doors' '0000a52a (/E-STEER Core/SubSystem Specifications/Application Functions/SF009A Thermal Duty Cycle Protection)' '#SF009A_285' 'true' 'REQ:  SF009A_285' '' } %GIDa_57703fab_89c6_46b9_a010_6a300dd59952"  SFunctionSpec=single y1 = Exp_f32(single u1)  ShowSpec=on
      settings: AttributesFormatString=%<MaskType>
  Gain : Gain  RequirementInfo="{'linktype_rmi_doors' '0000a52a (/E-STEER Core/SubSystem Specifications/Application Functions/SF009A Thermal Duty Cycle Protection)' '#SF009A_285' 'true' 'REQ:  SF009A_285' '' } %GIDa_c87ee9d0_4095_4a61_9d3d_879e8b6486a8"  Gain=-1
  Product1 : Product  RequirementInfo="{'linktype_rmi_doors' '0000a52a (/E-STEER Core/SubSystem Specifications/Application Functions/SF009A Thermal Duty Cycle Protection)' '#SF009A_285' 'true' 'REQ:  SF009A_285' '' } %GIDa_57d5ea56_1e55_4e31_b3e0_93aa11516aa8"  RndMeth=Zero
  Product2 : Product  RequirementInfo="{'linktype_rmi_doors' '0000a52a (/E-STEER Core/SubSystem Specifications/Application Functions/SF009A Thermal Duty Cycle Protection)' '#SF009A_285' 'true' 'REQ:  SF009A_285' '' } %GIDa_750dcb34_2abd_4894_bf5e_3b0e89131671"  Inputs=*/  RndMeth=Zero
  Tau : Constant  RequirementInfo="{'linktype_rmi_doors' '0000a52a (/E-STEER Core/SubSystem Specifications/Application Functions/SF009A Thermal Duty Cycle Protection)' '#SF009A_285' 'true' 'REQ:  SF009A_285' '' } %GIDa_b90e2574_3590_40ba_956f_a384e0479c3c"  Value=TAU4_SEC_F32
  FiltSV : Outport  RequirementInfo="{'linktype_rmi_doors' '0000a52a (/E-STEER Core/SubSystem Specifications/Application Functions/SF009A Thermal Duty Cycle Protection)' '#SF009A_285' 'true' 'REQ:  SF009A_285' '' } %GIDa_35520a0b_7ea8_496f_ac90_73364029aadc"
  wires:
  FiltSVOrg/1 -> Product1/2
  Product1/1 -> FiltSV/1
  IgnTimeOffSel/1 -> Gain/1
  Tau/1 -> Product2/2
  Exp_f32/1 -> Product1/1
  Product2/1 -> Exp_f32/1
  Gain/1 -> Product2/1

== system SF009A_DutyCycThermProtn/DutyCycThermProtn/DutyCycThermProtnInit1/PowerOnTasks/InputIgnOffTime/Filt5ExpDecay ==
  IgnTimeOffSel : Inport  RequirementInfo="{'linktype_rmi_doors' '0000a52a (/E-STEER Core/SubSystem Specifications/Application Functions/SF009A Thermal Duty Cycle Protection)' '#SF009A_285' 'true' 'REQ:  SF009A_285' '' } %GIDa_b90161fb_4064_45d7_9d6b_cab682484744"
  FiltSVOrg : Inport  RequirementInfo="{'linktype_rmi_doors' '0000a52a (/E-STEER Core/SubSystem Specifications/Application Functions/SF009A Thermal Duty Cycle Protection)' '#SF009A_285' 'true' 'REQ:  SF009A_285' '' } %GIDa_f17c0eee_319f_4b2a_a1b3_070a9180d2cb"  Port=2
  CopyRight2 : Subsystem  Description=|  mask(Copyright Information){none=on}
      | Copyright info block.                                               
      |                                                                     
      | Place copyright information at the top of every subsystem in design.
      mask prompts: none "No parameters"
      mask help: Place copyright information at the top of every subsystem in design.
      mask Display:
      | NxtrConf = 'Nexteer Confidential';
      | 
      | sys = bdroot; %handle for the current model ("system")
      | first = get_param(sys,'Created');
      | first = first(end-3:end);  %year is last four digits
      | 
      | last = get_param(sys,'LastModifiedDate');
      | if isempty(last)
      |     last = datestr(now,'yyyy');
      | else
      |     last = last(end-3:end);
      | end
      | 
      | if strcmp(first,last)
      |     fprintf('%s -- Copyright %s Nexteer',NxtrConf,first)
      | else
      |     fprintf('%s -- %s%s- %s Nexteer',NxtrConf,char(169),first,last)
      | end
  Exp_f32 : NxtrMath/Exp_f32  RequirementInfo="{'linktype_rmi_doors' '0000a52a (/E-STEER Core/SubSystem Specifications/Application Functions/SF009A Thermal Duty Cycle Protection)' '#SF009A_285' 'true' 'REQ:  SF009A_285' '' } %GIDa_aca0274c_5d2f_4959_ab19_73663ecd45f4"  SFunctionSpec=single y1 = Exp_f32(single u1)  ShowSpec=on
      settings: AttributesFormatString=%<MaskType>
  Gain : Gain  RequirementInfo="{'linktype_rmi_doors' '0000a52a (/E-STEER Core/SubSystem Specifications/Application Functions/SF009A Thermal Duty Cycle Protection)' '#SF009A_285' 'true' 'REQ:  SF009A_285' '' } %GIDa_4e414b39_97a9_4e9b_aa01_66e532f180aa"  Gain=-1
  Product1 : Product  RequirementInfo="{'linktype_rmi_doors' '0000a52a (/E-STEER Core/SubSystem Specifications/Application Functions/SF009A Thermal Duty Cycle Protection)' '#SF009A_285' 'true' 'REQ:  SF009A_285' '' } %GIDa_3ff6f461_99a4_4da1_aecf_e72e027f0494"  RndMeth=Zero
  Product2 : Product  RequirementInfo="{'linktype_rmi_doors' '0000a52a (/E-STEER Core/SubSystem Specifications/Application Functions/SF009A Thermal Duty Cycle Protection)' '#SF009A_285' 'true' 'REQ:  SF009A_285' '' } %GIDa_a1ba9507_d090_4b6b_9d20_3c1727d1ce95"  Inputs=*/  RndMeth=Zero
  Tau : Constant  RequirementInfo="{'linktype_rmi_doors' '0000a52a (/E-STEER Core/SubSystem Specifications/Application Functions/SF009A Thermal Duty Cycle Protection)' '#SF009A_285' 'true' 'REQ:  SF009A_285' '' } %GIDa_3c638df1_c7fd_4e50_a802_ff31d0fe74ad"  Value=TAU5_SEC_F32
  FiltSV : Outport  RequirementInfo="{'linktype_rmi_doors' '0000a52a (/E-STEER Core/SubSystem Specifications/Application Functions/SF009A Thermal Duty Cycle Protection)' '#SF009A_285' 'true' 'REQ:  SF009A_285' '' } %GIDa_34068f8f_8835_45d5_8e2c_de5fc32af880"
  wires:
  FiltSVOrg/1 -> Product1/2
  Product1/1 -> FiltSV/1
  IgnTimeOffSel/1 -> Gain/1
  Tau/1 -> Product2/2
  Exp_f32/1 -> Product1/1
  Product2/1 -> Exp_f32/1
  Gain/1 -> Product2/1

== system SF009A_DutyCycThermProtn/DutyCycThermProtn/DutyCycThermProtnInit1/PowerOnTasks/InputIgnOffTime/Filt6ExpDecay ==
  IgnTimeOffSel : Inport  RequirementInfo="{'linktype_rmi_doors' '0000a52a (/E-STEER Core/SubSystem Specifications/Application Functions/SF009A Thermal Duty Cycle Protection)' '#SF009A_285' 'true' 'REQ:  SF009A_285' '' } %GIDa_fdad97c5_2a7e_4b19_aee1_16e53b4fa469"
  FiltSVOrg : Inport  RequirementInfo="{'linktype_rmi_doors' '0000a52a (/E-STEER Core/SubSystem Specifications/Application Functions/SF009A Thermal Duty Cycle Protection)' '#SF009A_285' 'true' 'REQ:  SF009A_285' '' } %GIDa_62f56edd_175f_4c7b_815e_c7943bed403b"  Port=2
  CopyRight2 : Subsystem  Description=|  mask(Copyright Information){none=on}
      | Copyright info block.                                               
      |                                                                     
      | Place copyright information at the top of every subsystem in design.
      mask prompts: none "No parameters"
      mask help: Place copyright information at the top of every subsystem in design.
      mask Display:
      | NxtrConf = 'Nexteer Confidential';
      | 
      | sys = bdroot; %handle for the current model ("system")
      | first = get_param(sys,'Created');
      | first = first(end-3:end);  %year is last four digits
      | 
      | last = get_param(sys,'LastModifiedDate');
      | if isempty(last)
      |     last = datestr(now,'yyyy');
      | else
      |     last = last(end-3:end);
      | end
      | 
      | if strcmp(first,last)
      |     fprintf('%s -- Copyright %s Nexteer',NxtrConf,first)
      | else
      |     fprintf('%s -- %s%s- %s Nexteer',NxtrConf,char(169),first,last)
      | end
  Exp_f32 : NxtrMath/Exp_f32  RequirementInfo="{'linktype_rmi_doors' '0000a52a (/E-STEER Core/SubSystem Specifications/Application Functions/SF009A Thermal Duty Cycle Protection)' '#SF009A_285' 'true' 'REQ:  SF009A_285' '' } %GIDa_442b610e_7bae_4f5d_a580_07fd6a86bb9f"  SFunctionSpec=single y1 = Exp_f32(single u1)  ShowSpec=on
      settings: AttributesFormatString=%<MaskType>
  Gain : Gain  RequirementInfo="{'linktype_rmi_doors' '0000a52a (/E-STEER Core/SubSystem Specifications/Application Functions/SF009A Thermal Duty Cycle Protection)' '#SF009A_285' 'true' 'REQ:  SF009A_285' '' } %GIDa_b39b7229_baa0_4654_9a01_936ece545f12"  Gain=-1
  Product1 : Product  RequirementInfo="{'linktype_rmi_doors' '0000a52a (/E-STEER Core/SubSystem Specifications/Application Functions/SF009A Thermal Duty Cycle Protection)' '#SF009A_285' 'true' 'REQ:  SF009A_285' '' } %GIDa_63ecbc7b_6765_47a2_aab0_c4aabe4b6ba4"  RndMeth=Zero
  Product2 : Product  RequirementInfo="{'linktype_rmi_doors' '0000a52a (/E-STEER Core/SubSystem Specifications/Application Functions/SF009A Thermal Duty Cycle Protection)' '#SF009A_285' 'true' 'REQ:  SF009A_285' '' } %GIDa_7bd2ccc2_3f25_47c1_a9ea_e44af7634a29"  Inputs=*/  RndMeth=Zero
  Tau : Constant  RequirementInfo="{'linktype_rmi_doors' '0000a52a (/E-STEER Core/SubSystem Specifications/Application Functions/SF009A Thermal Duty Cycle Protection)' '#SF009A_285' 'true' 'REQ:  SF009A_285' '' } %GIDa_9b08b9e4_ef81_4b23_b03d_82f472a8b4ee"  Value=TAU6_SEC_F32
  FiltSV : Outport  RequirementInfo="{'linktype_rmi_doors' '0000a52a (/E-STEER Core/SubSystem Specifications/Application Functions/SF009A Thermal Duty Cycle Protection)' '#SF009A_285' 'true' 'REQ:  SF009A_285' '' } %GIDa_7a9019c6_2f75_4e61_ae74_87f156da8ec8"
  wires:
  FiltSVOrg/1 -> Product1/2
  Product1/1 -> FiltSV/1
  IgnTimeOffSel/1 -> Gain/1
  Tau/1 -> Product2/2
  Exp_f32/1 -> Product1/1
  Product2/1 -> Exp_f32/1
  Gain/1 -> Product2/1

== system SF009A_DutyCycThermProtn/DutyCycThermProtn/DutyCycThermProtnPer1/FiltSVReinit/VehTiVldDisabled/CopyRight2 ==

== system SF009A_DutyCycThermProtn/DutyCycThermProtn/DutyCycThermProtnPer1/FiltSVReinit/VehTiVldEnabled/CopyRight2 ==
